simulink model "mbed_nucleo_f446_AppShield"  (R2015a)
settings: Solver=FixedStepDiscrete  SolverMode=SingleTasking  StartTime=0.0  StopTime=10.0  FixedStep=1e-3  RelTol=1e-3
libraries: mbed_lib x12, simulink x4, mbed_spi_several x1, mbed_i2c_sensors x1
settings Model: Creator=oh  LastModifiedBy=oh
settings OptimizationCC: OptimizeModelRefInitCode=on  LifeSpan=1
settings HardwareCC: ProdLargestAtomicInteger=Long  ProdLargestAtomicFloat=Double  ProdEndianess=LittleEndian  ProdHWDeviceType=ARM Compatible->ARM Cortex
settings RTWCC: SystemTargetFile=mbed.tlc  TemplateMakefile=mbed.tmf  Description=Mbed Target (Embedded Target)  TargetLang=C++
settings CodeAppCC: IgnoreCustomStorageClasses=off
settings STFCustomTargetCC: CombineOutputUpdateFcns=on  SupportContinuousTime=off  SupportVariableSizeSignals=off  SystemTargetFile=mbed.tlc
settings ERTTargetCC: SupportContinuousTime=off  SupportVariableSizeSignals=off  ERTCustomFileTemplate=mbed_file_process.tlc

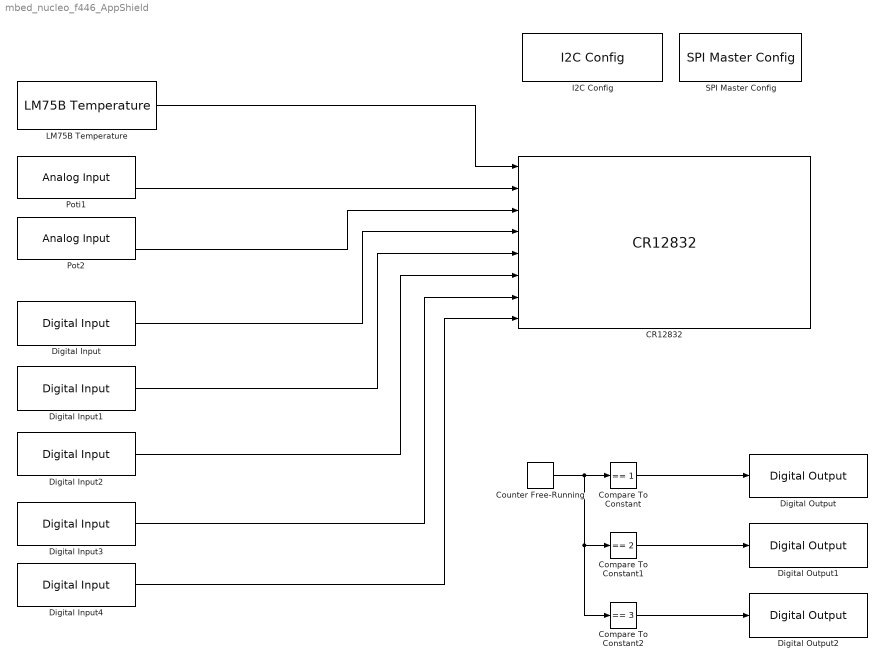
== system mbed_nucleo_f446_AppShield ==
  CR12832 : mbed_spi_several/CR12832  TypeOfInputs1={'single'}  NumberOfInputs1=1  Row1='Temperatur %f'  TypeOfInputs2={'single'}  NumberOfInputs2=1  Row2='Poti1 %f'  TypeOfInputs3={'single' 'uint8' 'uint8' 'uint8' 'uint8' 'uint8'}  NumberOfInputs3=6  Row3='Poti2 %f %hu %hu %hu %hu %hu'  SpiPort=1  CsPort=B  CsPin=6  ResPort=A  ResPin=6  A0Port=A  A0Pin=8  SampleTime=0.1
  Compare To Constant : simulink/Logic and Bit Operations/Compare To Constant  relop===  const=1  OutDataTypeStr=uint8
  Compare To Constant1 : simulink/Logic and Bit Operations/Compare To Constant  relop===  const=2  OutDataTypeStr=uint8
  Compare To Constant2 : simulink/Logic and Bit Operations/Compare To Constant  relop===  const=3  OutDataTypeStr=uint8
  Counter Free-Running : simulink/Sources/Counter Free-Running  NumBits=2  tsamp=0.1
  Digital Input : mbed_lib/GPIO/Digital Input  SParameter2=A  SParameter1=4  SParameter3=PullDefault  SampleTime=0.1
  Digital Input1 : mbed_lib/GPIO/Digital Input  SParameter2=B  SParameter1=0  SParameter3=PullDefault  SampleTime=0.1
  Digital Input2 : mbed_lib/GPIO/Digital Input  SParameter2=C  SParameter1=1  SParameter3=PullDefault  SampleTime=0.1
  Digital Input3 : mbed_lib/GPIO/Digital Input  SParameter2=C  SParameter1=0  SParameter3=PullDefault  SampleTime=0.1
  Digital Input4 : mbed_lib/GPIO/Digital Input  SParameter2=B  SParameter1=3  SParameter3=PullDefault  SampleTime=0.1
  Digital Output : mbed_lib/GPIO/Digital Output  SParameter2=A  SParameter1=10  SParameter3=PullDefault  SampleTime=-1
  Digital Output1 : mbed_lib/GPIO/Digital Output  SParameter2=A  SParameter1=9  SParameter3=PullDefault  SampleTime=-1
  Digital Output2 : mbed_lib/GPIO/Digital Output  SParameter2=C  SParameter1=7  SParameter3=PullDefault  SampleTime=-1
  I2C Config : mbed_lib/I2C/I2C Config  Priority=0  I2cPort=1  SParameter6=100000  SParameter2=B  SParameter3=9  SParameter4=B  SParameter5=8
  LM75B Temperature : mbed_i2c_sensors/LM75B Temperature  I2cPort=1  SampleTime=0.1
  Pot2 : mbed_lib/GPIO/Analog Input  SParameter2=A  SParameter1=1  SampleTime=0.1
  Poti1 : mbed_lib/GPIO/Analog Input  SParameter2=A  SParameter1=0  SampleTime=0.1
  SPI Master Config : mbed_lib/SPI/SPI Master Config  Priority=0  SpiPort=1  SpiFreq=100000  MosiPort=A  MosiPin=7  MisoPort=A  MisoPin=6  SclkPort=A  SclkPin=5
  wires:
  Poti1/2 -> CR12832/2
  Pot2/2 -> CR12832/3
  LM75B Temperature/1 -> CR12832/1
  Counter Free-Running/1 -> Compare To Constant2/1, Compare To Constant1/1, Compare To Constant/1
  Compare To Constant/1 -> Digital Output/1
  Compare To Constant1/1 -> Digital Output1/1
  Compare To Constant2/1 -> Digital Output2/1
  Digital Input/1 -> CR12832/4
  Digital Input1/1 -> CR12832/5
  Digital Input2/1 -> CR12832/6
  Digital Input3/1 -> CR12832/7
  Digital Input4/1 -> CR12832/8
